simulink model "industrial_45"  (R2021a)
settings: Solver=ode45  StartTime=0.0  StopTime=0.1  RelTol=1e-3
libraries: spsThyristorLib x6, spsGroundLib x1, spsSeriesRLCLoadLib x1, spsThreePhaseProgrammableVoltageSourceLib x1, spsVoltageMeasurementLib x1, spspowerguiLib x1
settings Model: Creator=Rohit  LastModifiedBy=Souvik Datta
settings SolverCC: AlgebraicLoopSolver=TrustRegion
settings DataIOCC: ReturnWorkspaceOutputs=off
settings DebuggingCC: SFMachineParentedDataDiag=warning  ArithmeticOperatorsInVariantConditions=warning
settings SFSimCC: SimUseLocalCustomCode=off  CustomCodeUndefinedFunction=UseInterfaceOnly
settings RTWCC: RTWUseLocalCustomCode=off

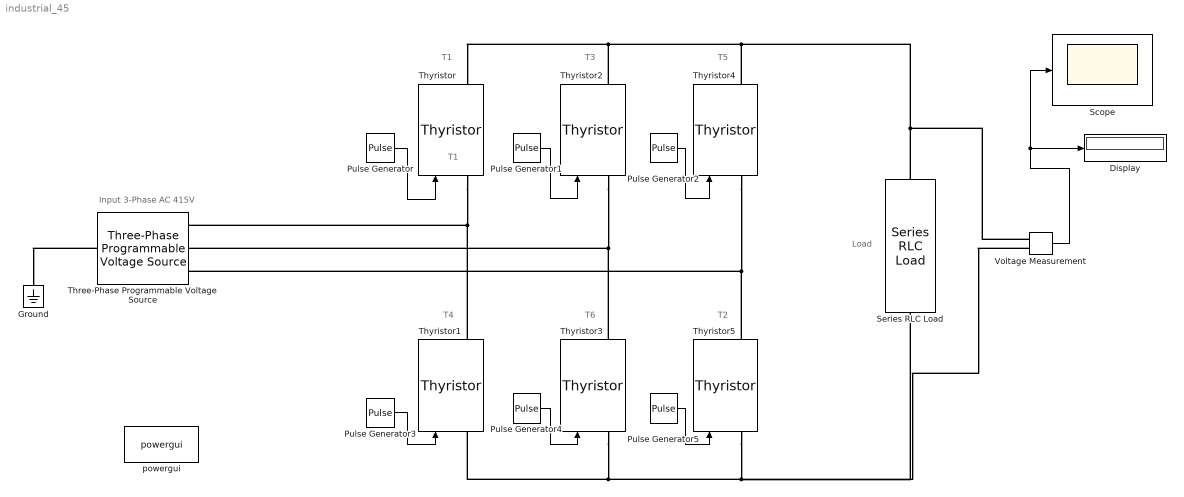
== system industrial_45 ==
  note: Input 3-Phase AC 415V
  note: T1
  note: T1
  note: T3
  note: T5
  note: T2
  note: T4
  note: T6
  note: Load
  Display : Display
  Ground : spsGroundLib/Ground  LConnTagsString=a
  Pulse Generator : DiscretePulseGenerator  PulseType=Time based  Amplitude=5  Period=20e-3  PulseWidth=35  PhaseDelay=2.5e-3
  Pulse Generator1 : DiscretePulseGenerator  PulseType=Time based  Amplitude=5  Period=20e-3  PulseWidth=35  PhaseDelay=9.16e-3
  Pulse Generator2 : DiscretePulseGenerator  PulseType=Time based  Amplitude=5  Period=20e-3  PulseWidth=35  PhaseDelay=15.8e-3
  Pulse Generator3 : DiscretePulseGenerator  PulseType=Time based  Amplitude=5  Period=20e-3  PulseWidth=35  PhaseDelay=12.5e-3
  Pulse Generator4 : DiscretePulseGenerator  PulseType=Time based  Amplitude=5  Period=20e-3  PulseWidth=35  PhaseDelay=19.16e-3
  Pulse Generator5 : DiscretePulseGenerator  PulseType=Time based  Amplitude=5  Period=20e-3  PulseWidth=35  PhaseDelay=25.8e-3
  Scope : Scope
  Series RLC Load : spsSeriesRLCLoadLib/Series RLC Load  LConnTagsString=a  RConnTagsString=__new0  NominalVoltage=415  NominalFrequency=50  ActivePower=1000  InductivePower=1732  CapacitivePower=0  Setx0=off  InitialVoltage=0  SetiL0=off  InitialCurrent=0  Measurements=None  LoadType=constant Z
  Three-Phase Programmable Voltage Source : spsThreePhaseProgrammableVoltageSourceLib/Three-Phase Programmable Voltage Source  PositiveSequence="[415  0 50]"  VariationEntity=None  VariationType=Table of time-amplitude pairs  VariationTypeAlt=Step  VariationStep=0.5  VariationRate=10  VariationMagnitude=0.3  VariationFrequency=2  VariationTiming=[1 2]  VariationPhaseA=off  Amplitudes=[1 0.8 1.2 1.0]  TimeValues=[0 0.1 0.15 0.2]  HarmonicGeneration=off  HarmonicA=[3 0.2 -25 0]  HarmonicB=[2 0.15 35 2]  Timing="[0.05  3]"  BusType=swing  Pref=0  Qref=0  Qmin=-inf  Qmax=inf
  Thyristor{,1..5} (6 alike) : spsThyristorLib/Thyristor  Ron=0.001  Lon=0  Vf=0.8  IC=0  Rs=500  Cs=250e-9  Measurements=on
  Voltage Measurement : spsVoltageMeasurementLib/Voltage Measurement  PhasorSimulation=off  OutputType=Complex  PSBequivalent=0
  powergui : spspowerguiLib/powergui  Priority=1  SimulationMode=Continuous  SampleTime=50e-6  frequency=60  Iterations=50  frequencyindice=50  Pbase=100e6  ErrMax=1e-4  UnitsV=kV  UnitsW=MW  buscounter=0  FunctionMessages=off  echomessages=off  EnableUseOfTLC=off  CurrentSourceSwitches=off  DisableSnubberDevices=off  DisableRonSwitches=off  DisableVfSwitches=off  DisplayEquations=off  AutomaticDiscreteSolvers=off  SolverType=Tustin/Backward Euler (TBE)  Interpol=off  ExternalGateDelay=off  methode=off  Ts=100  x0status=blocks  SPID=on  SwTol=0  HookPort=off  NonlinearTolerance=1e-4  nMaxIteration=100  ContinueOnMaxIteration=off  RestoreLinks=warning  ResistiveCurrentMeasurement=off  Frange=[0:2:500]  Ylog=off  Xlog=on  ShowGrid=off  save=off  variable=ZData  structure=0  ZoomFFT=off  StartTime=0.0  cycles=1  DisplayStyle=1  fundamental=60  FreqAxis=off  MaxFrequency=1000  frequencyindicesteady=1  RmsSteady=1  display=off
  wires:
  Pulse Generator2/1 -> Thyristor4/1
  Pulse Generator/1 -> Thyristor/1
  Pulse Generator4/1 -> Thyristor3/1
  Pulse Generator1/1 -> Thyristor2/1
  Pulse Generator3/1 -> Thyristor1/1
  Pulse Generator5/1 -> Thyristor5/1
  Voltage Measurement/1 -> Scope/1, Display/1
  connections:
  Three-Phase Programmable Voltage Source/LConn1 -- Ground/LConn1
  Thyristor1/RConn1 -- Thyristor/LConn1 -- Three-Phase Programmable Voltage Source/RConn1
  Thyristor3/RConn1 -- Thyristor2/LConn1 -- Three-Phase Programmable Voltage Source/RConn2
  Thyristor5/RConn1 -- Thyristor4/LConn1 -- Three-Phase Programmable Voltage Source/RConn3
  Series RLC Load/LConn1 -- Voltage Measurement/LConn1 -- Thyristor4/RConn1 -- Thyristor2/RConn1 -- Thyristor/RConn1
  Thyristor5/LConn1 -- Series RLC Load/RConn1 -- Voltage Measurement/LConn2 -- Thyristor3/LConn1 -- Thyristor1/LConn1
